simulink model "FinalYearSim_1D (1)"  (R2020b)
settings: Solver=VariableStepAuto  StartTime=0.0  StopTime=3  RelTol=1e-3
undefined symbols (not defined in the file): A, B, K1, K2, K3
settings Model: Creator=Debayan Das  LastModifiedBy=megsi
settings SFSimCC: CustomCodeUndefinedFunction=UseInterfaceOnly

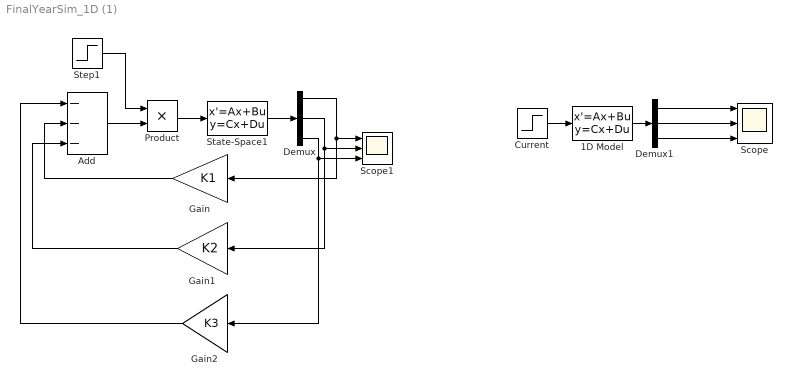
== system FinalYearSim_1D (1) ==
  1D Model : StateSpace  A=A  B=B  C=[1 0 0; 0 1 0; 0 0 1]  D=[0; 0; 0]  InitialCondition=[-pi/30; 0; 0]
  Add : Sum  Inputs=---
  Current : Step  Time=0  After=12  SampleTime=0
  Demux : Demux  Outputs=3
  Demux1 : Demux  Outputs=3
  Gain : Gain  Gain=K1
  Gain1 : Gain  Gain=K2
  Gain2 : Gain  Gain=K3
  Product : Product
  Scope : Scope  NumInputPorts=3
  Scope1 : Scope  NumInputPorts=3
  State-Space1 : StateSpace  A=A  B=B  C=[1 0 0; 0 1 0; 0 0 1]  D=[0; 0; 0]  InitialCondition=[-pi/30; 0; 0]
  Step1 : Step  Time=0  After=12  SampleTime=0
  wires:
  Step1/1 -> Product/1
  Demux/2 -> Scope1/2, Gain1/1
  Demux/3 -> Scope1/3, Gain2/1
  Demux/1 -> Scope1/1, Gain/1
  Gain/1 -> Add/2
  Gain1/1 -> Add/3
  Gain2/1 -> Add/1
  State-Space1/1 -> Demux/1
  Add/1 -> Product/2
  Product/1 -> State-Space1/1
  Current/1 -> 1D Model/1
  1D Model/1 -> Demux1/1
  Demux1/1 -> Scope/1
  Demux1/2 -> Scope/2
  Demux1/3 -> Scope/3
